simulink model "untitled"  (R2018b)
settings: Solver=VariableStepAuto  StartTime=0.0  StopTime=400  RelTol=1e-3
values from neighbouring files (symbols this model uses):
  g = 9.8    [aa.m]
  k = 1252*1000    (= 1252000)    [aa.m]
  M1 = 17*1000    (= 17000)    [aa.m]
  M2 = 754.2*1000    (= 754200)    [aa.m]
  mu = 0.02    [aa.m]
undefined symbols (not defined in the file or in its folder): sigbuilder_block, sth
libraries: simulink x1
settings Model: Creator=pkiop  LastModifiedBy=pkiop

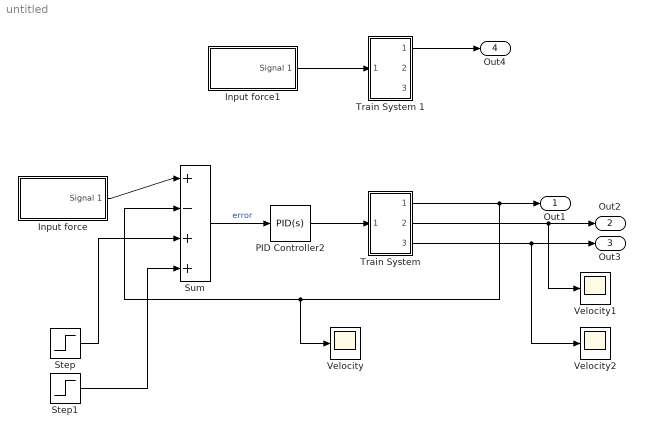
== system untitled ==
  Input force : Subsystem  Tag=STV Subsys  LoadFcn=sigbuilder_block('load');  StartFcn=sigbuilder_block('start');  StopFcn=sigbuilder_block('stop');  ClipboardFcn=sigbuilder_block('clipboard');  mask(Sigbuilder block){tuvar=[0:10]}
      mask help: Simulink:masks:SigbuilderBlock_MD
      mask init:
      | if ~strcmp(get_param(bdroot(gcbh),'SimulationStatus'),'stopped') tuvar = sigbuilder_block('maskInit'); end
      settings: CopyFcn=sigbuilder_block('copy');  DeleteFcn=sigbuilder_block('delete');  ModelCloseFcn=sigbuilder_block('modelClose');  PreSaveFcn=sigbuilder_block('preSave');  PauseFcn=sigbuilder_block('pause');  ContinueFcn=sigbuilder_block('continue');  NameChangeFcn=sigbuilder_block('namechange');  OpenFcn=sigbuilder_block('open',[437.6 199.2 550.4 400 ]);  CloseFcn=sigbuilder_block('close');
      mask Display: plot(0, 0, 100, 100,[2, 2, 32, 32, 2], [68, 8, 8, 68, 68],[32, 2], [38, 38], [32, 19, 2],[53, 60, 44], [32, 17, 17, 2],[16, 16, 31, 31]);txt = getActiveGroup(gcbh);text(2, 100, txt,'verticalAlignment', 'top');
  Input force1 : Subsystem  Tag=STV Subsys  LoadFcn=sigbuilder_block('load');  StartFcn=sigbuilder_block('start');  StopFcn=sigbuilder_block('stop');  ClipboardFcn=sigbuilder_block('clipboard');  mask(Sigbuilder block){tuvar=[0:10]}
      mask help: Simulink:masks:SigbuilderBlock_MD
      mask init:
      | if ~strcmp(get_param(bdroot(gcbh),'SimulationStatus'),'stopped') tuvar = sigbuilder_block('maskInit'); end
      settings: CopyFcn=sigbuilder_block('copy');  DeleteFcn=sigbuilder_block('delete');  ModelCloseFcn=sigbuilder_block('modelClose');  PreSaveFcn=sigbuilder_block('preSave');  PauseFcn=sigbuilder_block('pause');  ContinueFcn=sigbuilder_block('continue');  NameChangeFcn=sigbuilder_block('namechange');  OpenFcn=sigbuilder_block('open',[437.6 199.2 550.4 400 ]);  CloseFcn=sigbuilder_block('close');
      mask Display: plot(0, 0, 100, 100,[2, 2, 32, 32, 2], [68, 8, 8, 68, 68],[32, 2], [38, 38], [32, 19, 2],[53, 60, 44], [32, 17, 17, 2],[16, 16, 31, 31]);txt = getActiveGroup(gcbh);text(2, 100, txt,'verticalAlignment', 'top');
  PID Controller2 : simulink/Continuous/PID Controller  Controller=PID  Form=Parallel  TimeDomain=Continuous-time  SampleTime=-1  IntegratorMethod=Forward Euler  FilterMethod=Forward Euler  ControllerParametersSource=internal  P=0.000001  I=0.00305  D=0  UseFilter=on  N=100  TunerSelectOption=Transfer Function Based (PID Tuner App)  InitialConditionSource=internal  InitialConditionForIntegrator=0  InitialConditionForFilter=0  DifferentiatorICPrevScaledInput=0  ExternalReset=none  TrackingMode=off  Kt=1  LimitOutput=off  UpperSaturationLimit=inf  LowerSaturationLimit=-inf  LinearizeAsGain=on  AntiWindupMode=none  Kb=1  POutMin=[]  POutMax=[]  IOutMin=[]  IOutMax=[]  DOutMin=[]  DOutMax=[]  NOutMin=[]  NOutMax=[]  SumOutMin=[]  SumOutMax=[]  SaturationOutMin=[]  SaturationOutMax=[]  PParamMin=[]  PParamMax=[]  IParamMin=[]  IParamMax=[]  DParamMin=[]  DParamMax=[]  NParamMin=[]  NParamMax=[]  KbParamMin=[]  KbParamMax=[]  KtParamMin=[]  KtParamMax=[]  KbOutMin=[]  KbOutMax=[]  KtOutMin=[]  KtOutMax=[]  IntegratorOutMin=[]  IntegratorOutMax=[]  FilterOutMin=[]  FilterOutMax=[]  SumI1OutMin=[]  SumI1OutMax=[]  SumI2OutMin=[]  SumI2OutMax=[]  SumI3OutMin=[]  SumI3OutMax=[]  SumI4OutMin=[]  SumI4OutMax=[]  SumDOutMin=[]  SumDOutMax=[]  DifferentiatorOutMin=[]  DifferentiatorOutMax=[]  FilterDiffOutCoefMin=[]  FilterDiffOutCoefMax=[]  ReciprocalOutMin=[]  ReciprocalOutMax=[]  SumDenOutMin=[]  SumDenOutMax=[]  SumNumOutMin=[]  SumNumOutMax=[]  DivideOutMin=[]  DivideOutMax=[]  IntegratorContinuousStateAttributes=''  IntegratorStateMustResolveToSignalObject=off  IntegratorRTWStateStorageClass=Auto  FilterContinuousStateAttributes=''  FilterStateMustResolveToSignalObject=off  FilterRTWStateStorageClass=Auto  ParallelPVariant=InternalParameters  IdealPVariant=Disabled  IVariant=InternalParameters  DVariant=InternalParameters  IntegratorVariant=Continuous  SatVariant=Disabled  AWVariant=Passthrough  PCopyVariant=Disabled  TRVariant=Disabled  FdbkBlocksVariant=Forward  IdealPFdbkVariant=Disabled  SatFdbkVariant=Disabled  DerivativeFilterVariant=ContFilter  NVariant=InternalParameters  NCopyVariant=Disabled  FilterICVariant=InternalICsFilter  IntegratorICVariant=InternalICs  ExternalResetVariant=Disabled  TRSumVariant=Passthrough  SumFdbkVariant=Disabled  SumVariant=Sum_PID
  Step : Step  Time=500  After=(M1 + M2) * g * sth * (-1)  SampleTime=0
  Step1 : Step  Time=600  After=(M1 + M2) * g * sth  SampleTime=0
  Sum : Sum  Inputs=|+-++
  "Train System " : Subsystem
  Train System 1 : Subsystem
  Velocity : Scope
  Velocity1 : Scope
  Velocity2 : Scope
  Out1 : Outport
  Out2 : Outport  Port=2
  Out3 : Outport  Port=3
  Out4 : Outport  Port=4
  wires:
  "Train System "/2(Out2) -> Velocity1/1, Out2/1
  "Train System "/3(Out3) -> Velocity2/1, Out3/1
  "Train System "/1(Out1) -> Out1/1, Velocity/1, Sum/2
  Sum/1 -> PID Controller2/1  "error"
  Input force/1(Signal 1) -> Sum/1
  PID Controller2/1 -> "Train System "/1(In1)
  Step/1 -> Sum/3
  Step1/1 -> Sum/4
  Train System 1/1(Out1) -> Out4/1
  Input force1/1(Signal 1) -> Train System 1/1(In1)

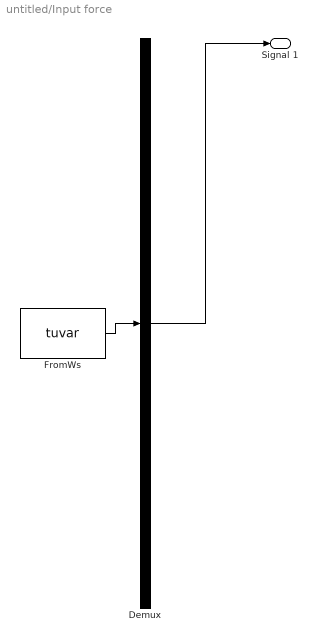
== system untitled/Input force ==
  Demux : Demux  Tag=STV Demux  Outputs=1
  FromWs : FromWorkspace  Tag=STV FromWs  VariableName=tuvar  SampleTime=0
      SigBuilderData=|
      | common.afterFinalStr = 'Extrapolate'
      | common.sampleTime = 0
      | dataSet.timeRange = [0 800]
      | dataSet.name = 'Group 1'
      | sbobj.Groups.Name = 'Group 1'
      | sbobj.Groups.Signals.Name = 'Signal 1'
      | sbobj.Groups.Signals.XData = [0 1.26 1.26 360 360 800]
      | sbobj.Groups.Signals.YData = [0 0 11100000 11100000 0 0]
      | sbobj.Groups.TimeRange = [0 800]
  Signal 1 : Outport  Tag=STV Outport
  wires:
  Demux/1 -> Signal 1/1
  FromWs/1 -> Demux/1

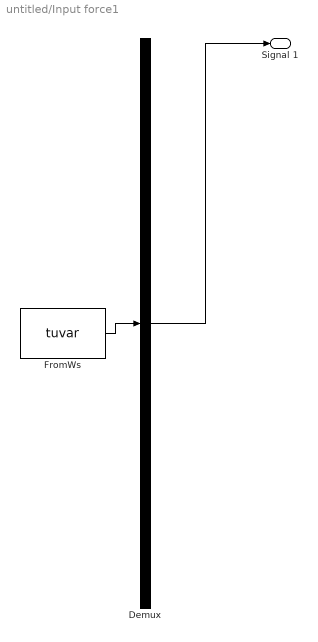
== system untitled/Input force1 ==
  Demux : Demux  Tag=STV Demux  Outputs=1
  FromWs : FromWorkspace  Tag=STV FromWs  VariableName=tuvar  SampleTime=0
      SigBuilderData=|
      | common.afterFinalStr = 'Extrapolate'
      | common.sampleTime = 0
      | dataSet.timeRange = [0 800]
      | dataSet.name = 'Group 1'
      | sbobj.Groups.Name = 'Group 1'
      | sbobj.Groups.Signals.Name = 'Signal 1'
      | sbobj.Groups.Signals.XData = [0 1.26 1.26 360 360 800]
      | sbobj.Groups.Signals.YData = [0 0 11100000 11100000 0 0]
      | sbobj.Groups.TimeRange = [0 800]
  Signal 1 : Outport  Tag=STV Outport
  wires:
  Demux/1 -> Signal 1/1
  FromWs/1 -> Demux/1

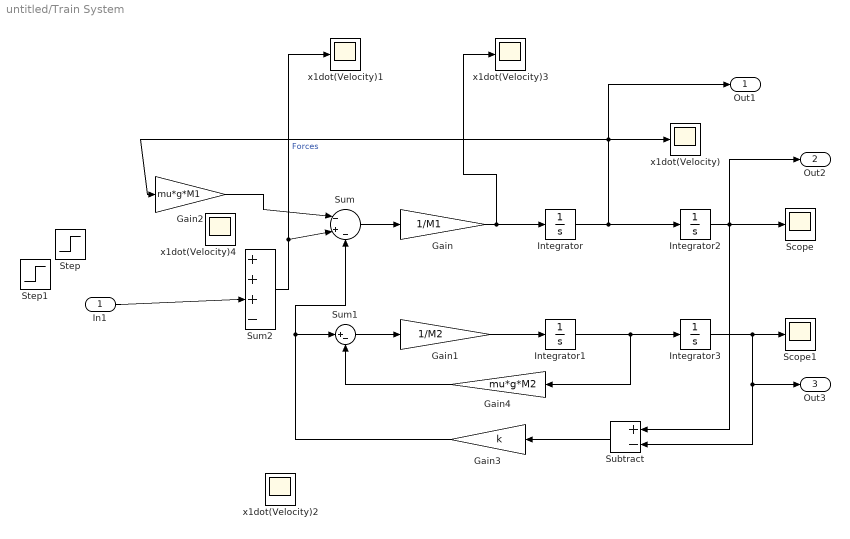
== system untitled/Train System  ==
  In1 : Inport
  Gain : Gain  Gain=1/M1
  Gain1 : Gain  Gain=1/M2
  Gain2 : Gain  Gain=mu*g*M1
  Gain3 : Gain  Gain=k
  Gain4 : Gain  Gain=mu*g*M2
  Integrator{,1..3} (4 alike) : Integrator
  Scope : Scope
  Scope1 : Scope
  Step : Step  Time=500  After=(M1 + M2) * g * sth * (-1)  SampleTime=0
  Step1 : Step  Time=600  After=(M1 + M2) * g * sth  SampleTime=0
  Subtract : Sum  Inputs=+-
  Sum : Sum  Inputs=|-+-
  Sum1 : Sum  Inputs=|+-
  Sum2 : Sum  Inputs=|+++-
  x1dot(Velocity){,1..4} (5 alike) : Scope
  Out1 : Outport
  Out2 : Outport  Port=2
  Out3 : Outport  Port=3
  wires:
  Integrator3/1 -> Out3/1, Subtract/2, Scope1/1
  Integrator2/1 -> Out2/1, Subtract/1, Scope/1
  Gain/1 -> x1dot(Velocity)3/1, Integrator/1
  Integrator/1 -> Out1/1, Gain2/1, x1dot(Velocity)/1, Integrator2/1
  Gain1/1 -> Integrator1/1
  Integrator1/1 -> Gain4/1, Integrator3/1
  Sum1/1 -> Gain1/1
  Sum2/1 -> x1dot(Velocity)1/1, Sum/2  "Forces"
  Subtract/1 -> Gain3/1
  Gain3/1 -> Sum/3, Sum1/1
  Gain4/1 -> Sum1/2
  Sum/1 -> Gain/1
  Gain2/1 -> Sum/1
  In1/1 -> Sum2/3

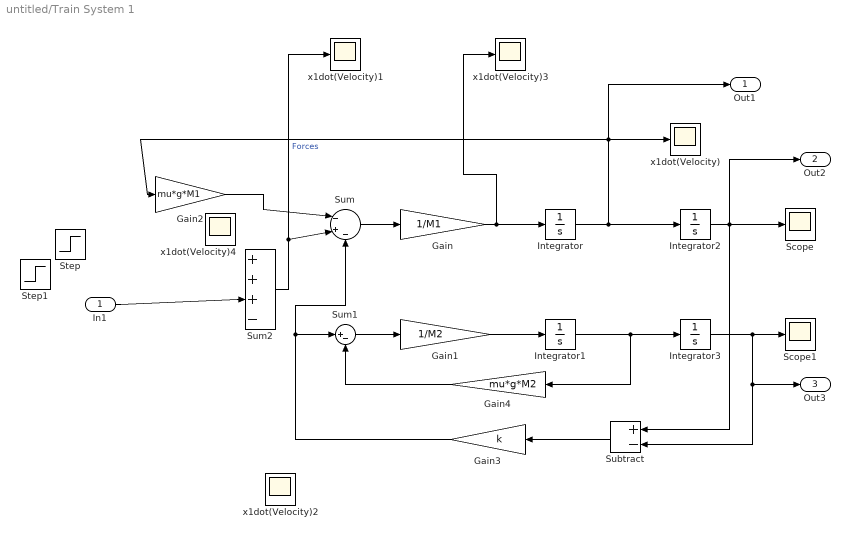
== system untitled/Train System 1 ==
  In1 : Inport
  Gain : Gain  Gain=1/M1
  Gain1 : Gain  Gain=1/M2
  Gain2 : Gain  Gain=mu*g*M1
  Gain3 : Gain  Gain=k
  Gain4 : Gain  Gain=mu*g*M2
  Integrator{,1..3} (4 alike) : Integrator
  Scope : Scope
  Scope1 : Scope
  Step : Step  Time=500  After=(M1 + M2) * g * sth * (-1)  SampleTime=0
  Step1 : Step  Time=600  After=(M1 + M2) * g * sth  SampleTime=0
  Subtract : Sum  Inputs=+-
  Sum : Sum  Inputs=|-+-
  Sum1 : Sum  Inputs=|+-
  Sum2 : Sum  Inputs=|+++-
  x1dot(Velocity){,1..4} (5 alike) : Scope
  Out1 : Outport
  Out2 : Outport  Port=2
  Out3 : Outport  Port=3
  wires:
  Integrator3/1 -> Out3/1, Subtract/2, Scope1/1
  Integrator2/1 -> Out2/1, Subtract/1, Scope/1
  Gain/1 -> x1dot(Velocity)3/1, Integrator/1
  Integrator/1 -> Out1/1, Gain2/1, x1dot(Velocity)/1, Integrator2/1
  Gain1/1 -> Integrator1/1
  Integrator1/1 -> Gain4/1, Integrator3/1
  Sum1/1 -> Gain1/1
  Sum2/1 -> x1dot(Velocity)1/1, Sum/2  "Forces"
  Subtract/1 -> Gain3/1
  Gain3/1 -> Sum/3, Sum1/1
  Gain4/1 -> Sum1/2
  Sum/1 -> Gain/1
  Gain2/1 -> Sum/1
  In1/1 -> Sum2/3
